simulink model "HSX_PPS_series0226_2"  (R2023b)
settings: Solver=VariableStepAuto  StartTime=0.0  StopTime=10  RelTol=1e-3
undefined symbols (not defined in the file): Kanti, Ki, Kp, LHSX, Ra, RHSX, Tsamp, Vf
libraries: spsVoltageMeasurementLib x39, spsControlledVoltageSourceLib x32, spsDCMachineLib x32, spsSeriesRLCBranchLib x8, spsCurrentMeasurementLib x6, spsGroundLib x3, spsIdealSwitchLib x2, spsMosfetLib x2, spsPWMGenerator2LevelLib x1, spsDCVoltageSourceLib x1, spsDiodeLib x1, spsVariableRatioTransformerLib x1
(part 1 of 2)
settings Model: Creator=Hyeongmeen  LastModifiedBy=Hyeongmeen

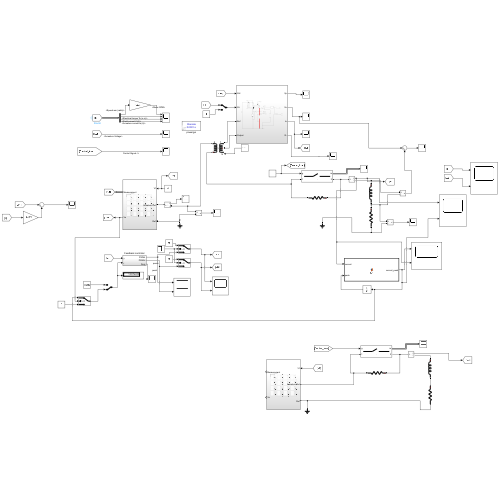
[thumbnail: Simulink's stored preview of the top-level diagram]
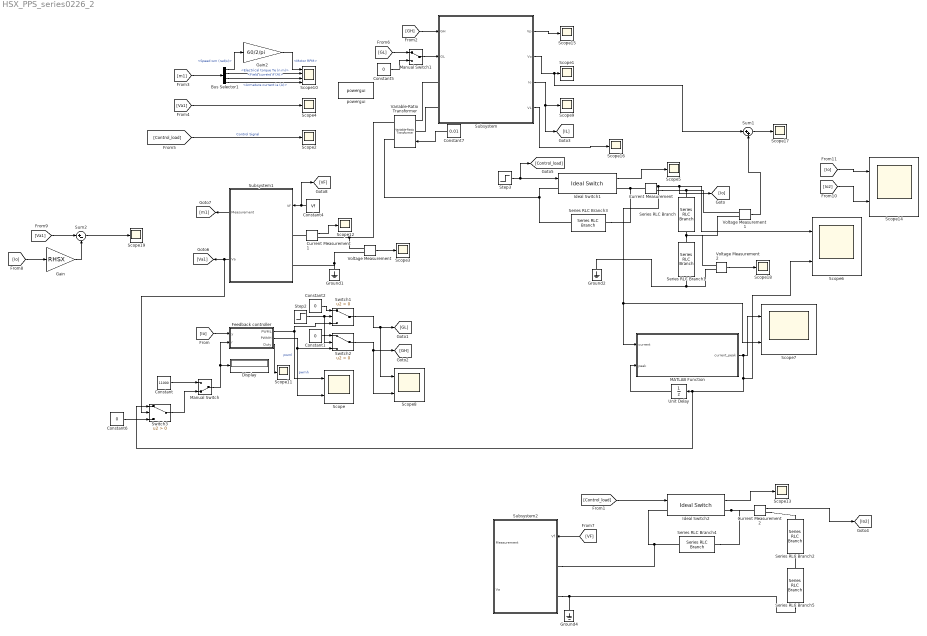
== system HSX_PPS_series0226_2 ==
  Bus Selector1 : BusSelector  OutputSignals=Speed wm (rad/s),Electrical torque Te (n m),Field current if (A),Armature current ia (A)
  Constant : Constant  Value=11000
  Constant{1..2,5..6} (4 alike) : Constant  Value=0
  Constant4 : Constant  Value=Vf
  Constant7 : Constant  Value=0.01
  Current Measurement : spsCurrentMeasurementLib/Current Measurement  PhasorSimulation=off  OutputType=Complex  PSBequivalent=0
  Current Measurement1 : spsCurrentMeasurementLib/Current Measurement  PhasorSimulation=off  OutputType=Complex  PSBequivalent=0
  Current Measurement2 : spsCurrentMeasurementLib/Current Measurement  PhasorSimulation=off  OutputType=Complex  PSBequivalent=0
  Display : Display
  Feedback controller : Subsystem
  Gain : Gain  Gain=RHSX
  Gain2 : Gain  Gain=60/2/pi
  Ground1 : spsGroundLib/Ground  LConnTagsString=a
  Ground2 : spsGroundLib/Ground  LConnTagsString=a
  Ground4 : spsGroundLib/Ground  LConnTagsString=a
  Ideal Switch1 : spsIdealSwitchLib/Ideal Switch  Ron=0.01  Lon=0  IC=0  Rs=1e6  Cs=0  Measurements=on
  Ideal Switch2 : spsIdealSwitchLib/Ideal Switch  Ron=0.01  Lon=0  IC=0  Rs=1e6  Cs=0  Measurements=on
  MATLAB Function : MATLAB Function  TreatAsAtomicUnit=on
  Manual Switch : ManualSwitch  CurrentSetting=0
  Manual Switch1 : ManualSwitch
  Scope{,6..8,14} (5 alike) : Scope  NumInputPorts=2
  Scope{1..5,9,11..13,15..19} (14 alike) : Scope
  Scope10 : Scope  NumInputPorts=4
  Series RLC Branch : spsSeriesRLCBranchLib/Series RLC Branch  LConnTagsString=__new0  RConnTagsString=__new0  BranchType=L  Resistance=RHSX  Inductance=LHSX  SetiL0=off  InitialCurrent=0  Capacitance=1e-6  Setx0=off  InitialVoltage=0  Measurements=None
  Series RLC Branch1 : spsSeriesRLCBranchLib/Series RLC Branch  LConnTagsString=__new0  RConnTagsString=__new0  BranchType=R  Resistance=RHSX  Inductance=LHSX  SetiL0=off  InitialCurrent=0  Capacitance=1e-6  Setx0=off  InitialVoltage=0  Measurements=None
  Series RLC Branch2 : spsSeriesRLCBranchLib/Series RLC Branch  LConnTagsString=__new0  RConnTagsString=__new0  BranchType=L  Resistance=RHSX  Inductance=LHSX  SetiL0=off  InitialCurrent=0  Capacitance=1e-6  Setx0=off  InitialVoltage=0  Measurements=None
  Series RLC Branch3 : spsSeriesRLCBranchLib/Series RLC Branch  LConnTagsString=__new0  RConnTagsString=__new0  BranchType=R  Resistance=1e8  Inductance=0  SetiL0=off  InitialCurrent=0  Capacitance=1e-6  Setx0=off  InitialVoltage=0  Measurements=None
  Series RLC Branch4 : spsSeriesRLCBranchLib/Series RLC Branch  LConnTagsString=__new0  RConnTagsString=__new0  BranchType=R  Resistance=1e8  Inductance=0  SetiL0=off  InitialCurrent=0  Capacitance=1e-6  Setx0=off  InitialVoltage=0  Measurements=None
  Series RLC Branch5 : spsSeriesRLCBranchLib/Series RLC Branch  LConnTagsString=__new0  RConnTagsString=__new0  BranchType=R  Resistance=RHSX  Inductance=LHSX  SetiL0=off  InitialCurrent=0  Capacitance=1e-6  Setx0=off  InitialVoltage=0  Measurements=None
  Step2 : Step  Time=5  Before=1  After=0  SampleTime=0  VectorParams1D=off  ZeroCross=off
  Step3 : Step  Time=5  SampleTime=0  VectorParams1D=off  ZeroCross=off
  Subsystem : Subsystem
  Subsystem1 : Subsystem
  Subsystem2 : Subsystem
  Sum1 : Sum  Inputs=|++
  Sum2 : Sum  Inputs=|+-
  Switch1 : Switch  Criteria=u2 > Threshold  SaturateOnIntegerOverflow=off  InputSameDT=off
  Switch2 : Switch  Criteria=u2 > Threshold  SaturateOnIntegerOverflow=off  InputSameDT=off
  Switch3 : Switch  Criteria=u2 > Threshold  SaturateOnIntegerOverflow=off  InputSameDT=off
  Unit Delay : UnitDelay  SampleTime=-1  HasFrameUpgradeWarning=on
  Variable-Ratio Transformer : spsVariableRatioTransformerLib/Variable-Ratio Transformer
      settings: LibrarySourceBlock=|
      | sps_lib/Passives/Variable-Ratio
      | Transformer
  Voltage Measurement : spsVoltageMeasurementLib/Voltage Measurement  PhasorSimulation=off  OutputType=Complex  PSBequivalent=0
  Voltage Measurement1 : spsVoltageMeasurementLib/Voltage Measurement  PhasorSimulation=off  OutputType=Complex  PSBequivalent=0
  Voltage Measurement2 : spsVoltageMeasurementLib/Voltage Measurement  PhasorSimulation=off  OutputType=Complex  PSBequivalent=0
  powergui : sps_lib/powergui  Priority=1  SimulationMode=Discrete  SampleTime=Tsamp  frequency=60  Iterations=50  frequencyindice=0  Pbase=100e6  ErrMax=1e-4  UnitsV=kV  UnitsW=MW  buscounter=0  FunctionMessages=off  echomessages=off  EnableUseOfTLC=off  CurrentSourceSwitches=off  DisableSnubberDevices=off  DisableRonSwitches=off  DisableVfSwitches=off  DisplayEquations=off  AutomaticDiscreteSolvers=off  SolverType=Tustin/Backward Euler (TBE)  Interpol=off  ExternalGateDelay=off  methode=off  Ts=100  x0status=blocks  SPID=on  SwTol=0  HookPort=off  NonlinearTolerance=1e-4  nMaxIteration=100  ContinueOnMaxIteration=off  RestoreLinks=warning  ResistiveCurrentMeasurement=off  Frange=[0:2:500]  Ylog=off  Xlog=on  ShowGrid=off  save=off  variable=ZData  structure=0  ZoomFFT=off  StartTime=0.0  cycles=1  DisplayStyle=1  fundamental=60  FreqAxis=off  MaxFrequency=1000  frequencyindicesteady=1  RmsSteady=1  display=off
  wires:
  Bus Selector1/1 -> Gain2/1  "<Speed wm (rad/s)>"
  Bus Selector1/4 -> Scope10/4  "<Armature current ia (A)>"
  Bus Selector1/2 -> Scope10/2  "<Electrical torque Te (n m)>"
  Gain2/1 -> Scope10/1  "<Motor RPM>"
  Bus Selector1/3 -> Scope10/3  "<Field current if (A)>"
  [m1] -> Bus Selector1/1
  Step3/1 -> [Control_load], Ideal Switch1/1
  Step2/1 -> Switch2/2, Switch1/2
  Feedback controller/2(PWMH) -> Switch2/3, Scope/2  "pwmh"
  Feedback controller/1(PWML) -> Scope/1, Switch1/3  "pwml"
  Constant2/1 -> Switch1/1
  Constant1/1 -> Switch2/1
  [Control_load] -> Scope2/1  "Control Signal"
  [Va1] -> Scope4/1
  Subsystem1/2(Va) -> Switch3/2, [Va1]
  Subsystem1/1(Measurement) -> [m1]
  Constant4/1 -> [VF], Subsystem1/1(Vf)
  Ideal Switch1/1 -> Scope5/1
  Current Measurement/1 -> Scope7/2, MATLAB Function/1(current), [Io], Scope6/1
  Unit Delay/1 -> MATLAB Function/2(peak)
  Switch1/1 -> Scope8/1, [GL]
  Switch2/1 -> Scope8/2, [GH]
  Subsystem/2(Vo) -> Sum1/1, Scope1/1
  Voltage Measurement/1 -> Scope3/1
  Subsystem/3(Io) -> [IL], Scope9/1
  Manual Switch1/1 -> Subsystem/2(GL)
  [Io] -> Feedback controller/1(y)
  Feedback controller/3(Duty) -> Scope11/1
  Constant/1 -> Manual Switch/1
  Manual Switch/1 -> Display/1, Feedback controller/2(r)
  [GH] -> Subsystem/1(GH)
  [GL] -> Manual Switch1/1
  Constant5/1 -> Manual Switch1/2
  MATLAB Function/1(current_peak) -> Scope6/2, Switch3/1, Unit Delay/1, Scope7/1
  Switch3/1 -> Manual Switch/2
  Constant6/1 -> Switch3/3
  Subsystem/1(Vp) -> Scope15/1
  Subsystem/4(VL) -> Scope16/1
  Voltage Measurement1/1 -> Sum1/2
  Sum1/1 -> Scope17/1
  Voltage Measurement2/1 -> Scope18/1
  [Va1] -> Sum2/1
  [Io] -> Gain/1
  Gain/1 -> Sum2/2
  Sum2/1 -> Scope19/1
  Current Measurement1/1 -> Scope12/1
  Constant7/1 -> Variable-Ratio Transformer/1
  Ideal Switch2/1 -> Scope13/1
  [Control_load] -> Ideal Switch2/1
  [VF] -> Subsystem2/1(Vf)
  Current Measurement2/1 -> [Io2]
  [Io] -> Scope14/1
  [Io2] -> Scope14/2
  connections:
  Series RLC Branch3/LConn1 -- Current Measurement/LConn1 -- Ideal Switch1/RConn1
  Ground1/LConn1 -- Voltage Measurement/LConn2 -- Subsystem1/LConn2
  Current Measurement/RConn1 -- Voltage Measurement1/LConn1 -- Series RLC Branch/LConn1
  Voltage Measurement/LConn1 -- Variable-Ratio Transformer/RConn2 -- Current Measurement1/RConn1
  Ground2/LConn1 -- Voltage Measurement2/LConn2 -- Series RLC Branch1/RConn1
  Series RLC Branch/RConn1 -- Voltage Measurement2/LConn1 -- Voltage Measurement1/LConn2 -- Series RLC Branch1/LConn1
  Subsystem/LConn1 -- Variable-Ratio Transformer/LConn2
  Current Measurement1/LConn1 -- Subsystem1/LConn1
  Ideal Switch1/LConn1 -- Variable-Ratio Transformer/RConn1 -- Series RLC Branch3/RConn1
  Subsystem/LConn2 -- Variable-Ratio Transformer/LConn1
  Ideal Switch2/LConn1 -- Subsystem2/LConn1 -- Series RLC Branch4/RConn1
  Current Measurement2/RConn1 -- Series RLC Branch2/LConn1
  Ideal Switch2/RConn1 -- Series RLC Branch4/LConn1 -- Current Measurement2/LConn1
  Subsystem2/LConn2 -- Series RLC Branch5/RConn1 -- Ground4/LConn1
  Series RLC Branch5/LConn1 -- Series RLC Branch2/RConn1

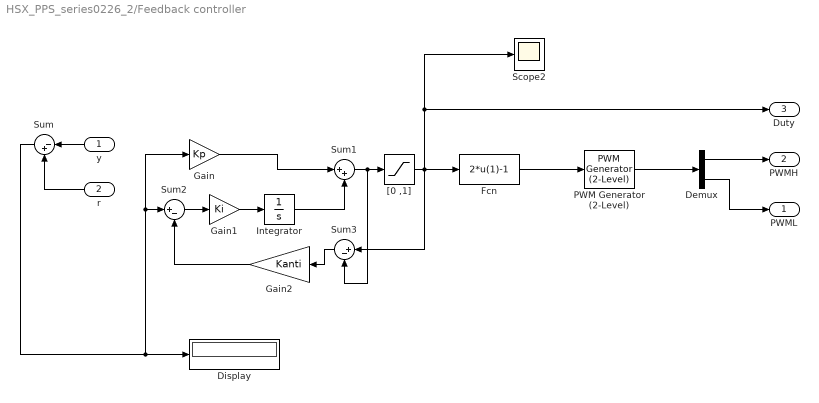
== system HSX_PPS_series0226_2/Feedback controller ==
  y : Inport
  r : Inport  Port=2
  Demux : Demux  Outputs=2
  Display : Display
  Fcn : Fcn  Expr=2*u(1)-1
  Gain : Gain  Gain=Kp
  Gain1 : Gain  Gain=Ki
  Gain2 : Gain  Gain=Kanti
  Integrator : Integrator
  PWM Generator (2-Level) : spsPWMGenerator2LevelLib/PWM Generator (2-Level)  ModulatorType=Single-phase half-bridge (2 pulses)  ModulatorMode=Unsynchronized  Fc=10000  Pc=90  nF=27  MinMax="[ -1  1 ]"  SamplingTechnique=Natural  ModulatingSignals=off  m=0.8  Freq=60  Phase=0  Ts=0  ShowCarrierOutport=off
  Scope2 : Scope
  Sum : Sum  Inputs=|-+  InputSameDT=on  SaturateOnIntegerOverflow=on  OutDataTypeStr=Inherit: Same as first input
  Sum1 : Sum  Inputs=|++
  Sum2 : Sum  Inputs=|+-
  Sum3 : Sum  Inputs=|+-
  "[0 ,1]" : Saturate  UpperLimit=1  LowerLimit=0
  PWML : Outport  VectorParamsAs1DForOutWhenUnconnected=off
  PWMH : Outport  Port=2  VectorParamsAs1DForOutWhenUnconnected=off
  Duty : Outport  Port=3  VectorParamsAs1DForOutWhenUnconnected=off
  wires:
  Sum/1 -> Display/1, Gain/1, Sum2/1
  y/1 -> Sum/1
  r/1 -> Sum/2
  "[0 ,1]"/1 -> Sum3/1, Fcn/1, Scope2/1, Duty/1
  Fcn/1 -> PWM Generator (2-Level)/1
  PWM Generator (2-Level)/1 -> Demux/1
  Demux/1 -> PWMH/1
  Demux/2 -> PWML/1
  Gain1/1 -> Integrator/1
  Sum1/1 -> Sum3/2, "[0 ,1]"/1
  Gain/1 -> Sum1/1
  Integrator/1 -> Sum1/2
  Sum2/1 -> Gain1/1
  Sum3/1 -> Gain2/1
  Gain2/1 -> Sum2/2

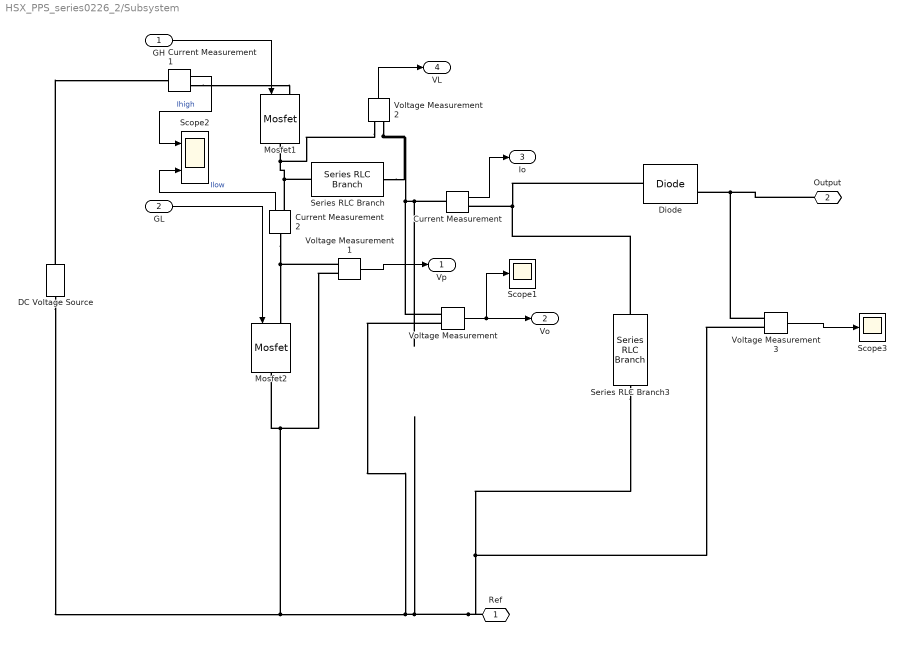
== system HSX_PPS_series0226_2/Subsystem ==
  GH : Inport
  GL : Inport  Port=2
  Current Measurement : spsCurrentMeasurementLib/Current Measurement  PhasorSimulation=off  OutputType=Complex  PSBequivalent=0
  Current Measurement1 : spsCurrentMeasurementLib/Current Measurement  PhasorSimulation=off  OutputType=Complex  PSBequivalent=0
  Current Measurement2 : spsCurrentMeasurementLib/Current Measurement  PhasorSimulation=off  OutputType=Complex  PSBequivalent=0
  DC Voltage Source : spsDCVoltageSourceLib/DC Voltage Source  Amplitude=2000  Measurements=None
  Diode : spsDiodeLib/Diode  Ron=0.001  Lon=0  Vf=0.8  IC=0  UseSnubber=0  Rs=500  Cs=250e-9  Measurements=on
  Mosfet1 : spsMosfetLib/Mosfet  Ron=0.00001  Lon=0  Rd=0.01  Vfd=0.8  IC=0  Rs=1e5  Cs=inf  Measurements=off
  Mosfet2 : spsMosfetLib/Mosfet  Ron=0.00001  Lon=0  Rd=0.01  Vfd=0.8  IC=0  Rs=1e5  Cs=inf  Measurements=off
  Scope1 : Scope
  Scope2 : Scope  NumInputPorts=2
  Scope3 : Scope
  Series RLC Branch : spsSeriesRLCBranchLib/Series RLC Branch  LConnTagsString=__new0  RConnTagsString=__new0  BranchType=L  Resistance=RHSX  Inductance=0.0001  SetiL0=off  InitialCurrent=0  Capacitance=1e-6  Setx0=off  InitialVoltage=0  Measurements=None
  Series RLC Branch3 : spsSeriesRLCBranchLib/Series RLC Branch  LConnTagsString=__new0  RConnTagsString=__new0  BranchType=R  Resistance=1e8  Inductance=0  SetiL0=off  InitialCurrent=0  Capacitance=1e-6  Setx0=off  InitialVoltage=0  Measurements=None
  Voltage Measurement{,1..3} (4 alike) : spsVoltageMeasurementLib/Voltage Measurement  PhasorSimulation=off  OutputType=Complex  PSBequivalent=0
  Ref : PMIOPort  Side=Left
  Output : PMIOPort  Port=2  Side=Left
  Vp : Outport
  Vo : Outport  Port=2
  Io : Outport  Port=3
  VL : Outport  Port=4
  wires:
  Voltage Measurement/1 -> Vo/1, Scope1/1
  Voltage Measurement1/1 -> Vp/1
  GL/1 -> Mosfet2/1
  GH/1 -> Mosfet1/1
  Current Measurement/1 -> Io/1
  Current Measurement1/1 -> Scope2/1  "Ihigh"
  Current Measurement2/1 -> Scope2/2  "Ilow"
  Voltage Measurement2/1 -> VL/1
  Voltage Measurement3/1 -> Scope3/1
  connections:
  Current Measurement2/RConn1 -- Series RLC Branch/LConn1 -- Voltage Measurement2/LConn1 -- Mosfet1/RConn1
  Ref/RConn1 -- Voltage Measurement3/LConn2 -- Series RLC Branch3/LConn1 -- Voltage Measurement/LConn2 -- Voltage Measurement1/LConn2 -- Mosfet2/RConn1 -- DC Voltage Source/LConn1
  Series RLC Branch3/RConn1 -- Diode/LConn1 -- Current Measurement/RConn1
  DC Voltage Source/RConn1 -- Current Measurement1/LConn1
  Current Measurement1/RConn1 -- Mosfet1/LConn1
  Voltage Measurement1/LConn1 -- Current Measurement2/LConn1 -- Mosfet2/LConn1
  Voltage Measurement2/LConn2 -- Series RLC Branch/RConn1 -- Voltage Measurement/LConn1 -- Current Measurement/LConn1
  Output/RConn1 -- Voltage Measurement3/LConn1 -- Diode/RConn1

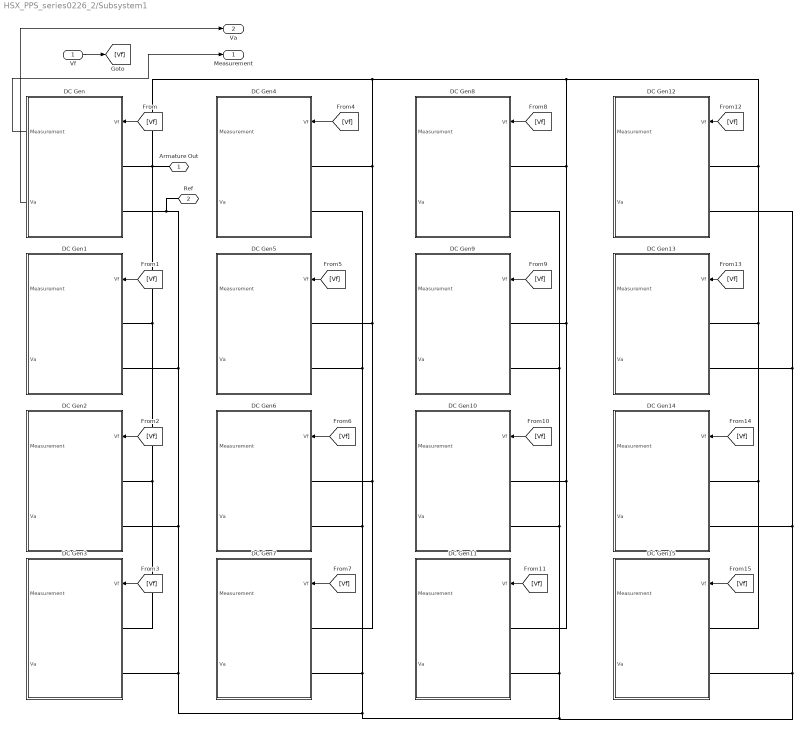
== system HSX_PPS_series0226_2/Subsystem1 ==
  Vf : Inport
  DC Gen : Subsystem
  DC Gen1 : Subsystem
  DC Gen10 : Subsystem
  DC Gen11 : Subsystem
  DC Gen12 : Subsystem
  DC Gen13 : Subsystem
  DC Gen14 : Subsystem
  DC Gen15 : Subsystem
  DC Gen2 : Subsystem
  DC Gen3 : Subsystem
  DC Gen4 : Subsystem
  DC Gen5 : Subsystem
  DC Gen6 : Subsystem
  DC Gen7 : Subsystem
  DC Gen8 : Subsystem
  DC Gen9 : Subsystem
  Armature Out : PMIOPort  Side=Left
  Ref : PMIOPort  Port=2  Side=Left
  Measurement : Outport
  Va : Outport  Port=2
  wires:
  Vf/1 -> [Vf]
  [Vf] -> DC Gen/1(Vf)
  [Vf] -> DC Gen1/1(Vf)
  [Vf] -> DC Gen2/1(Vf)
  [Vf] -> DC Gen3/1(Vf)
  [Vf] -> DC Gen4/1(Vf)
  [Vf] -> DC Gen5/1(Vf)
  [Vf] -> DC Gen6/1(Vf)
  [Vf] -> DC Gen7/1(Vf)
  [Vf] -> DC Gen8/1(Vf)
  [Vf] -> DC Gen9/1(Vf)
  [Vf] -> DC Gen10/1(Vf)
  [Vf] -> DC Gen11/1(Vf)
  [Vf] -> DC Gen12/1(Vf)
  [Vf] -> DC Gen13/1(Vf)
  [Vf] -> DC Gen14/1(Vf)
  [Vf] -> DC Gen15/1(Vf)
  DC Gen/1(Measurement) -> Measurement/1
  DC Gen/2(Va) -> Va/1
  connections:
  DC Gen11/LConn1 -- DC Gen10/LConn1 -- DC Gen9/LConn1 -- DC Gen8/LConn1 -- DC Gen7/LConn1 -- DC Gen6/LConn1 -- DC Gen5/LConn1 -- DC Gen4/LConn1 -- DC Gen1/LConn1 -- DC Gen2/LConn1 -- DC Gen3/LConn1 -- DC Gen/LConn1 -- Armature Out/RConn1 -- DC Gen12/LConn1 -- DC Gen13/LConn1 -- DC Gen14/LConn1 -- DC Gen15/LConn1
  DC Gen8/LConn2 -- DC Gen9/LConn2 -- DC Gen10/LConn2 -- DC Gen11/LConn2 -- DC Gen4/LConn2 -- DC Gen5/LConn2 -- DC Gen6/LConn2 -- DC Gen7/LConn2 -- DC Gen3/LConn2 -- DC Gen1/LConn2 -- Ref/RConn1 -- DC Gen/LConn2 -- DC Gen2/LConn2 -- DC Gen15/LConn2 -- DC Gen12/LConn2 -- DC Gen13/LConn2 -- DC Gen14/LConn2

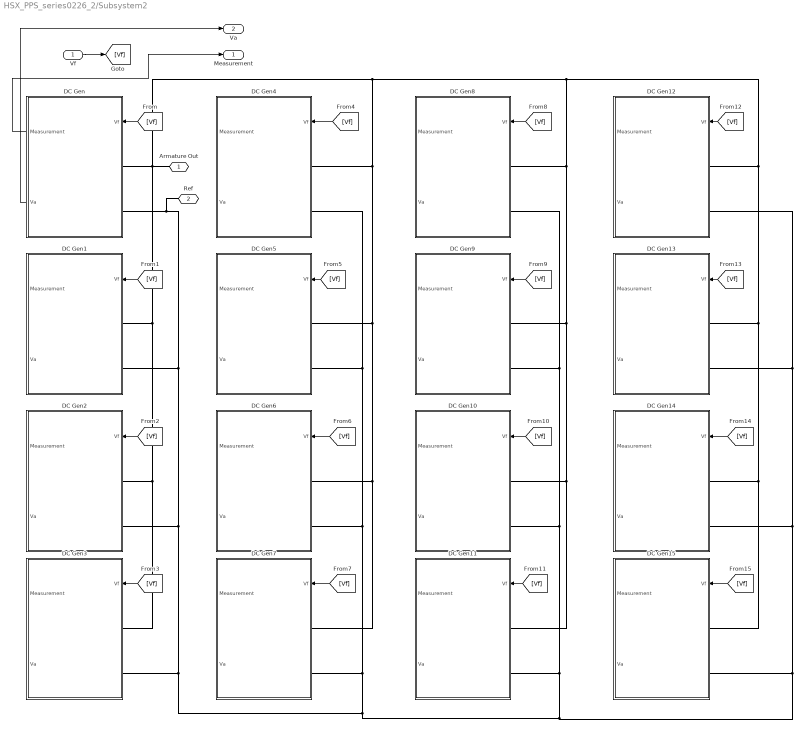
== system HSX_PPS_series0226_2/Subsystem2 ==
  Vf : Inport
  DC Gen : Subsystem
  DC Gen1 : Subsystem
  DC Gen10 : Subsystem
  DC Gen11 : Subsystem
  DC Gen12 : Subsystem
  DC Gen13 : Subsystem
  DC Gen14 : Subsystem
  DC Gen15 : Subsystem
  DC Gen2 : Subsystem
  DC Gen3 : Subsystem
  DC Gen4 : Subsystem
  DC Gen5 : Subsystem
  DC Gen6 : Subsystem
  DC Gen7 : Subsystem
  DC Gen8 : Subsystem
  DC Gen9 : Subsystem
  Armature Out : PMIOPort  Side=Left
  Ref : PMIOPort  Port=2  Side=Left
  Measurement : Outport
  Va : Outport  Port=2
  wires:
  Vf/1 -> [Vf]
  [Vf] -> DC Gen/1(Vf)
  [Vf] -> DC Gen1/1(Vf)
  [Vf] -> DC Gen2/1(Vf)
  [Vf] -> DC Gen3/1(Vf)
  [Vf] -> DC Gen4/1(Vf)
  [Vf] -> DC Gen5/1(Vf)
  [Vf] -> DC Gen6/1(Vf)
  [Vf] -> DC Gen7/1(Vf)
  [Vf] -> DC Gen8/1(Vf)
  [Vf] -> DC Gen9/1(Vf)
  [Vf] -> DC Gen10/1(Vf)
  [Vf] -> DC Gen11/1(Vf)
  [Vf] -> DC Gen12/1(Vf)
  [Vf] -> DC Gen13/1(Vf)
  [Vf] -> DC Gen14/1(Vf)
  [Vf] -> DC Gen15/1(Vf)
  DC Gen/1(Measurement) -> Measurement/1
  DC Gen/2(Va) -> Va/1
  connections:
  DC Gen11/LConn1 -- DC Gen10/LConn1 -- DC Gen9/LConn1 -- DC Gen8/LConn1 -- DC Gen7/LConn1 -- DC Gen6/LConn1 -- DC Gen5/LConn1 -- DC Gen4/LConn1 -- DC Gen1/LConn1 -- DC Gen2/LConn1 -- DC Gen3/LConn1 -- DC Gen/LConn1 -- Armature Out/RConn1 -- DC Gen12/LConn1 -- DC Gen13/LConn1 -- DC Gen14/LConn1 -- DC Gen15/LConn1
  DC Gen8/LConn2 -- DC Gen9/LConn2 -- DC Gen10/LConn2 -- DC Gen11/LConn2 -- DC Gen4/LConn2 -- DC Gen5/LConn2 -- DC Gen6/LConn2 -- DC Gen7/LConn2 -- DC Gen3/LConn2 -- DC Gen1/LConn2 -- Ref/RConn1 -- DC Gen/LConn2 -- DC Gen2/LConn2 -- DC Gen15/LConn2 -- DC Gen12/LConn2 -- DC Gen13/LConn2 -- DC Gen14/LConn2

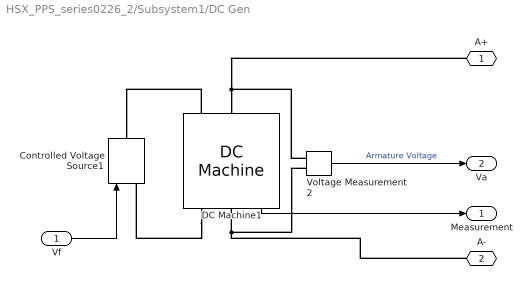
== system HSX_PPS_series0226_2/Subsystem1/DC Gen ==
  Vf : Inport
  Controlled Voltage Source1 : spsControlledVoltageSourceLib/Controlled Voltage Source  Initialize=on  Source_Type=DC  Amplitude=0  Phase=0  Frequency=0  Measurements=Voltage
  DC Machine1 : spsDCMachineLib/DC Machine  PresetModel=No  MechanicalLoad=Torque TL  FieldType=Wound  ShowDetailedParameters=on  MeasurementBus=off  RLa="[Ra  0.002]"  RLf=[0.0054 0.0125]  Laf=Laf  MachineConstant=Torque constant (N.m/A)  Ke=1.8  Kt=1.8  J=137  Bm=0  Tf=0  w0=w_initial  Ifinit=0  TsPowergui=0  TsBlock=-1
  Voltage Measurement2 : spsVoltageMeasurementLib/Voltage Measurement  PhasorSimulation=off  OutputType=Complex  PSBequivalent=0
  A+ : PMIOPort  Side=Left
  A- : PMIOPort  Port=2  Side=Left
  Measurement : Outport
  Va : Outport  Port=2
  wires:
  DC Machine1/1 -> Measurement/1
  Vf/1 -> Controlled Voltage Source1/1
  Voltage Measurement2/1 -> Va/1  "Armature Voltage"
  connections:
  Voltage Measurement2/LConn1 -- A+/RConn1 -- DC Machine1/LConn1
  A-/RConn1 -- Voltage Measurement2/LConn2 -- DC Machine1/RConn1
  DC Machine1/LConn2 -- Controlled Voltage Source1/RConn1
  DC Machine1/RConn2 -- Controlled Voltage Source1/LConn1

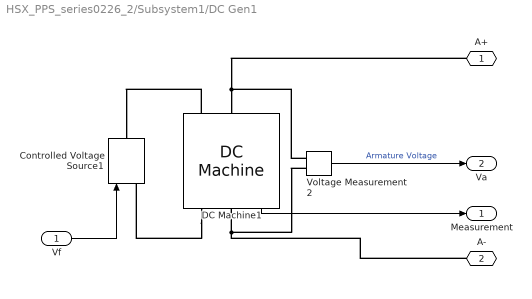
== system HSX_PPS_series0226_2/Subsystem1/DC Gen1 ==
  Vf : Inport
  Controlled Voltage Source1 : spsControlledVoltageSourceLib/Controlled Voltage Source  Initialize=on  Source_Type=DC  Amplitude=0  Phase=0  Frequency=0  Measurements=Voltage
  DC Machine1 : spsDCMachineLib/DC Machine  PresetModel=No  MechanicalLoad=Torque TL  FieldType=Wound  ShowDetailedParameters=on  MeasurementBus=off  RLa="[Ra  0.002]"  RLf=[0.0054 0.0125]  Laf=Laf  MachineConstant=Torque constant (N.m/A)  Ke=1.8  Kt=1.8  J=137  Bm=0  Tf=0  w0=w_initial  Ifinit=0  TsPowergui=0  TsBlock=-1
  Voltage Measurement2 : spsVoltageMeasurementLib/Voltage Measurement  PhasorSimulation=off  OutputType=Complex  PSBequivalent=0
  A+ : PMIOPort  Side=Left
  A- : PMIOPort  Port=2  Side=Left
  Measurement : Outport
  Va : Outport  Port=2
  wires:
  DC Machine1/1 -> Measurement/1
  Vf/1 -> Controlled Voltage Source1/1
  Voltage Measurement2/1 -> Va/1  "Armature Voltage"
  connections:
  Voltage Measurement2/LConn1 -- A+/RConn1 -- DC Machine1/LConn1
  A-/RConn1 -- Voltage Measurement2/LConn2 -- DC Machine1/RConn1
  DC Machine1/LConn2 -- Controlled Voltage Source1/RConn1
  DC Machine1/RConn2 -- Controlled Voltage Source1/LConn1

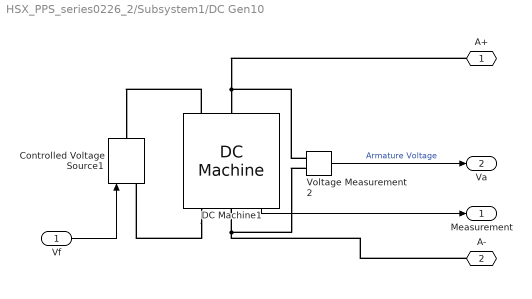
== system HSX_PPS_series0226_2/Subsystem1/DC Gen10 ==
  Vf : Inport
  Controlled Voltage Source1 : spsControlledVoltageSourceLib/Controlled Voltage Source  Initialize=on  Source_Type=DC  Amplitude=0  Phase=0  Frequency=0  Measurements=Voltage
  DC Machine1 : spsDCMachineLib/DC Machine  PresetModel=No  MechanicalLoad=Torque TL  FieldType=Wound  ShowDetailedParameters=on  MeasurementBus=off  RLa="[Ra  0.002]"  RLf=[0.0054 0.0125]  Laf=Laf  MachineConstant=Torque constant (N.m/A)  Ke=1.8  Kt=1.8  J=137  Bm=0  Tf=0  w0=w_initial  Ifinit=0  TsPowergui=0  TsBlock=-1
  Voltage Measurement2 : spsVoltageMeasurementLib/Voltage Measurement  PhasorSimulation=off  OutputType=Complex  PSBequivalent=0
  A+ : PMIOPort  Side=Left
  A- : PMIOPort  Port=2  Side=Left
  Measurement : Outport
  Va : Outport  Port=2
  wires:
  DC Machine1/1 -> Measurement/1
  Vf/1 -> Controlled Voltage Source1/1
  Voltage Measurement2/1 -> Va/1  "Armature Voltage"
  connections:
  Voltage Measurement2/LConn1 -- A+/RConn1 -- DC Machine1/LConn1
  A-/RConn1 -- Voltage Measurement2/LConn2 -- DC Machine1/RConn1
  DC Machine1/LConn2 -- Controlled Voltage Source1/RConn1
  DC Machine1/RConn2 -- Controlled Voltage Source1/LConn1

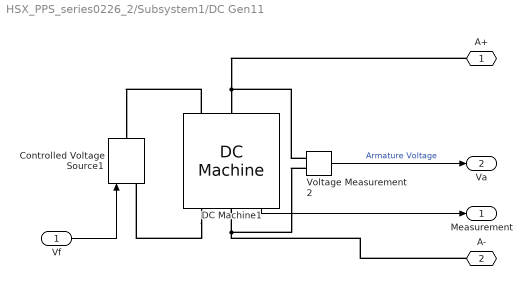
== system HSX_PPS_series0226_2/Subsystem1/DC Gen11 ==
  Vf : Inport
  Controlled Voltage Source1 : spsControlledVoltageSourceLib/Controlled Voltage Source  Initialize=on  Source_Type=DC  Amplitude=0  Phase=0  Frequency=0  Measurements=Voltage
  DC Machine1 : spsDCMachineLib/DC Machine  PresetModel=No  MechanicalLoad=Torque TL  FieldType=Wound  ShowDetailedParameters=on  MeasurementBus=off  RLa="[Ra  0.002]"  RLf=[0.0054 0.0125]  Laf=Laf  MachineConstant=Torque constant (N.m/A)  Ke=1.8  Kt=1.8  J=137  Bm=0  Tf=0  w0=w_initial  Ifinit=0  TsPowergui=0  TsBlock=-1
  Voltage Measurement2 : spsVoltageMeasurementLib/Voltage Measurement  PhasorSimulation=off  OutputType=Complex  PSBequivalent=0
  A+ : PMIOPort  Side=Left
  A- : PMIOPort  Port=2  Side=Left
  Measurement : Outport
  Va : Outport  Port=2
  wires:
  DC Machine1/1 -> Measurement/1
  Vf/1 -> Controlled Voltage Source1/1
  Voltage Measurement2/1 -> Va/1  "Armature Voltage"
  connections:
  Voltage Measurement2/LConn1 -- A+/RConn1 -- DC Machine1/LConn1
  A-/RConn1 -- Voltage Measurement2/LConn2 -- DC Machine1/RConn1
  DC Machine1/LConn2 -- Controlled Voltage Source1/RConn1
  DC Machine1/RConn2 -- Controlled Voltage Source1/LConn1

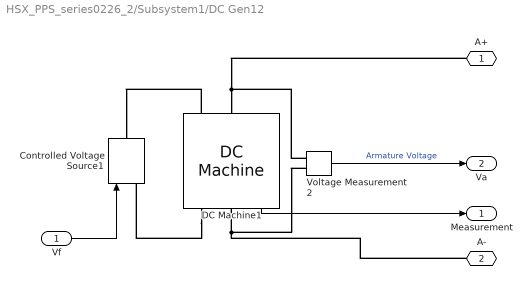
== system HSX_PPS_series0226_2/Subsystem1/DC Gen12 ==
  Vf : Inport
  Controlled Voltage Source1 : spsControlledVoltageSourceLib/Controlled Voltage Source  Initialize=on  Source_Type=DC  Amplitude=0  Phase=0  Frequency=0  Measurements=Voltage
  DC Machine1 : spsDCMachineLib/DC Machine  PresetModel=No  MechanicalLoad=Torque TL  FieldType=Wound  ShowDetailedParameters=on  MeasurementBus=off  RLa="[Ra  0.002]"  RLf=[0.0054 0.0125]  Laf=Laf  MachineConstant=Torque constant (N.m/A)  Ke=1.8  Kt=1.8  J=137  Bm=0  Tf=0  w0=w_initial  Ifinit=0  TsPowergui=0  TsBlock=-1
  Voltage Measurement2 : spsVoltageMeasurementLib/Voltage Measurement  PhasorSimulation=off  OutputType=Complex  PSBequivalent=0
  A+ : PMIOPort  Side=Left
  A- : PMIOPort  Port=2  Side=Left
  Measurement : Outport
  Va : Outport  Port=2
  wires:
  DC Machine1/1 -> Measurement/1
  Vf/1 -> Controlled Voltage Source1/1
  Voltage Measurement2/1 -> Va/1  "Armature Voltage"
  connections:
  Voltage Measurement2/LConn1 -- A+/RConn1 -- DC Machine1/LConn1
  A-/RConn1 -- Voltage Measurement2/LConn2 -- DC Machine1/RConn1
  DC Machine1/LConn2 -- Controlled Voltage Source1/RConn1
  DC Machine1/RConn2 -- Controlled Voltage Source1/LConn1

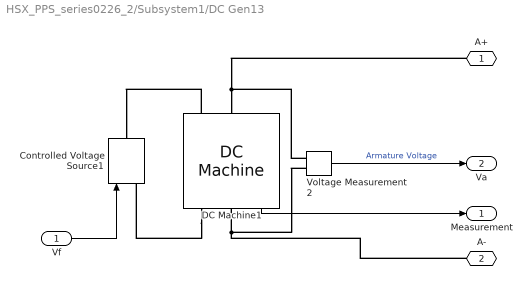
== system HSX_PPS_series0226_2/Subsystem1/DC Gen13 ==
  Vf : Inport
  Controlled Voltage Source1 : spsControlledVoltageSourceLib/Controlled Voltage Source  Initialize=on  Source_Type=DC  Amplitude=0  Phase=0  Frequency=0  Measurements=Voltage
  DC Machine1 : spsDCMachineLib/DC Machine  PresetModel=No  MechanicalLoad=Torque TL  FieldType=Wound  ShowDetailedParameters=on  MeasurementBus=off  RLa="[Ra  0.002]"  RLf=[0.0054 0.0125]  Laf=Laf  MachineConstant=Torque constant (N.m/A)  Ke=1.8  Kt=1.8  J=137  Bm=0  Tf=0  w0=w_initial  Ifinit=0  TsPowergui=0  TsBlock=-1
  Voltage Measurement2 : spsVoltageMeasurementLib/Voltage Measurement  PhasorSimulation=off  OutputType=Complex  PSBequivalent=0
  A+ : PMIOPort  Side=Left
  A- : PMIOPort  Port=2  Side=Left
  Measurement : Outport
  Va : Outport  Port=2
  wires:
  DC Machine1/1 -> Measurement/1
  Vf/1 -> Controlled Voltage Source1/1
  Voltage Measurement2/1 -> Va/1  "Armature Voltage"
  connections:
  Voltage Measurement2/LConn1 -- A+/RConn1 -- DC Machine1/LConn1
  A-/RConn1 -- Voltage Measurement2/LConn2 -- DC Machine1/RConn1
  DC Machine1/LConn2 -- Controlled Voltage Source1/RConn1
  DC Machine1/RConn2 -- Controlled Voltage Source1/LConn1

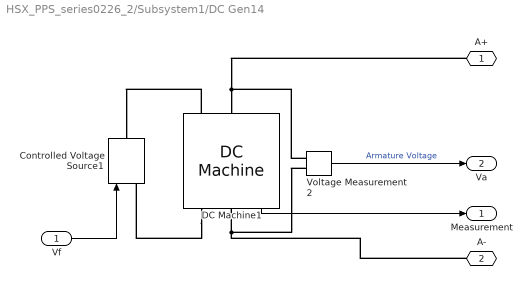
== system HSX_PPS_series0226_2/Subsystem1/DC Gen14 ==
  Vf : Inport
  Controlled Voltage Source1 : spsControlledVoltageSourceLib/Controlled Voltage Source  Initialize=on  Source_Type=DC  Amplitude=0  Phase=0  Frequency=0  Measurements=Voltage
  DC Machine1 : spsDCMachineLib/DC Machine  PresetModel=No  MechanicalLoad=Torque TL  FieldType=Wound  ShowDetailedParameters=on  MeasurementBus=off  RLa="[Ra  0.002]"  RLf=[0.0054 0.0125]  Laf=Laf  MachineConstant=Torque constant (N.m/A)  Ke=1.8  Kt=1.8  J=137  Bm=0  Tf=0  w0=w_initial  Ifinit=0  TsPowergui=0  TsBlock=-1
  Voltage Measurement2 : spsVoltageMeasurementLib/Voltage Measurement  PhasorSimulation=off  OutputType=Complex  PSBequivalent=0
  A+ : PMIOPort  Side=Left
  A- : PMIOPort  Port=2  Side=Left
  Measurement : Outport
  Va : Outport  Port=2
  wires:
  DC Machine1/1 -> Measurement/1
  Vf/1 -> Controlled Voltage Source1/1
  Voltage Measurement2/1 -> Va/1  "Armature Voltage"
  connections:
  Voltage Measurement2/LConn1 -- A+/RConn1 -- DC Machine1/LConn1
  A-/RConn1 -- Voltage Measurement2/LConn2 -- DC Machine1/RConn1
  DC Machine1/LConn2 -- Controlled Voltage Source1/RConn1
  DC Machine1/RConn2 -- Controlled Voltage Source1/LConn1

== system HSX_PPS_series0226_2/Subsystem1/DC Gen15 ==
  Vf : Inport
  Controlled Voltage Source1 : spsControlledVoltageSourceLib/Controlled Voltage Source  Initialize=on  Source_Type=DC  Amplitude=0  Phase=0  Frequency=0  Measurements=Voltage
  DC Machine1 : spsDCMachineLib/DC Machine  PresetModel=No  MechanicalLoad=Torque TL  FieldType=Wound  ShowDetailedParameters=on  MeasurementBus=off  RLa="[Ra  0.002]"  RLf=[0.0054 0.0125]  Laf=Laf  MachineConstant=Torque constant (N.m/A)  Ke=1.8  Kt=1.8  J=137  Bm=0  Tf=0  w0=w_initial  Ifinit=0  TsPowergui=0  TsBlock=-1
  Voltage Measurement2 : spsVoltageMeasurementLib/Voltage Measurement  PhasorSimulation=off  OutputType=Complex  PSBequivalent=0
  A+ : PMIOPort  Side=Left
  A- : PMIOPort  Port=2  Side=Left
  Measurement : Outport
  Va : Outport  Port=2
  wires:
  DC Machine1/1 -> Measurement/1
  Vf/1 -> Controlled Voltage Source1/1
  Voltage Measurement2/1 -> Va/1  "Armature Voltage"
  connections:
  Voltage Measurement2/LConn1 -- A+/RConn1 -- DC Machine1/LConn1
  A-/RConn1 -- Voltage Measurement2/LConn2 -- DC Machine1/RConn1
  DC Machine1/LConn2 -- Controlled Voltage Source1/RConn1
  DC Machine1/RConn2 -- Controlled Voltage Source1/LConn1

== system HSX_PPS_series0226_2/Subsystem1/DC Gen2 ==
  Vf : Inport
  Controlled Voltage Source1 : spsControlledVoltageSourceLib/Controlled Voltage Source  Initialize=on  Source_Type=DC  Amplitude=0  Phase=0  Frequency=0  Measurements=Voltage
  DC Machine1 : spsDCMachineLib/DC Machine  PresetModel=No  MechanicalLoad=Torque TL  FieldType=Wound  ShowDetailedParameters=on  MeasurementBus=off  RLa="[Ra  0.002]"  RLf=[0.0054 0.0125]  Laf=Laf  MachineConstant=Torque constant (N.m/A)  Ke=1.8  Kt=1.8  J=137  Bm=0  Tf=0  w0=w_initial  Ifinit=0  TsPowergui=0  TsBlock=-1
  Voltage Measurement2 : spsVoltageMeasurementLib/Voltage Measurement  PhasorSimulation=off  OutputType=Complex  PSBequivalent=0
  A+ : PMIOPort  Side=Left
  A- : PMIOPort  Port=2  Side=Left
  Measurement : Outport
  Va : Outport  Port=2
  wires:
  DC Machine1/1 -> Measurement/1
  Vf/1 -> Controlled Voltage Source1/1
  Voltage Measurement2/1 -> Va/1  "Armature Voltage"
  connections:
  Voltage Measurement2/LConn1 -- A+/RConn1 -- DC Machine1/LConn1
  A-/RConn1 -- Voltage Measurement2/LConn2 -- DC Machine1/RConn1
  DC Machine1/LConn2 -- Controlled Voltage Source1/RConn1
  DC Machine1/RConn2 -- Controlled Voltage Source1/LConn1

== system HSX_PPS_series0226_2/Subsystem1/DC Gen3 ==
  Vf : Inport
  Controlled Voltage Source1 : spsControlledVoltageSourceLib/Controlled Voltage Source  Initialize=on  Source_Type=DC  Amplitude=0  Phase=0  Frequency=0  Measurements=Voltage
  DC Machine1 : spsDCMachineLib/DC Machine  PresetModel=No  MechanicalLoad=Torque TL  FieldType=Wound  ShowDetailedParameters=on  MeasurementBus=off  RLa="[Ra  0.002]"  RLf=[0.0054 0.0125]  Laf=Laf  MachineConstant=Torque constant (N.m/A)  Ke=1.8  Kt=1.8  J=137  Bm=0  Tf=0  w0=w_initial  Ifinit=0  TsPowergui=0  TsBlock=-1
  Voltage Measurement2 : spsVoltageMeasurementLib/Voltage Measurement  PhasorSimulation=off  OutputType=Complex  PSBequivalent=0
  A+ : PMIOPort  Side=Left
  A- : PMIOPort  Port=2  Side=Left
  Measurement : Outport
  Va : Outport  Port=2
  wires:
  DC Machine1/1 -> Measurement/1
  Vf/1 -> Controlled Voltage Source1/1
  Voltage Measurement2/1 -> Va/1  "Armature Voltage"
  connections:
  Voltage Measurement2/LConn1 -- A+/RConn1 -- DC Machine1/LConn1
  A-/RConn1 -- Voltage Measurement2/LConn2 -- DC Machine1/RConn1
  DC Machine1/LConn2 -- Controlled Voltage Source1/RConn1
  DC Machine1/RConn2 -- Controlled Voltage Source1/LConn1

== system HSX_PPS_series0226_2/Subsystem1/DC Gen4 ==
  Vf : Inport
  Controlled Voltage Source1 : spsControlledVoltageSourceLib/Controlled Voltage Source  Initialize=on  Source_Type=DC  Amplitude=0  Phase=0  Frequency=0  Measurements=Voltage
  DC Machine1 : spsDCMachineLib/DC Machine  PresetModel=No  MechanicalLoad=Torque TL  FieldType=Wound  ShowDetailedParameters=on  MeasurementBus=off  RLa="[Ra  0.002]"  RLf=[0.0054 0.0125]  Laf=Laf  MachineConstant=Torque constant (N.m/A)  Ke=1.8  Kt=1.8  J=137  Bm=0  Tf=0  w0=w_initial  Ifinit=0  TsPowergui=0  TsBlock=-1
  Voltage Measurement2 : spsVoltageMeasurementLib/Voltage Measurement  PhasorSimulation=off  OutputType=Complex  PSBequivalent=0
  A+ : PMIOPort  Side=Left
  A- : PMIOPort  Port=2  Side=Left
  Measurement : Outport
  Va : Outport  Port=2
  wires:
  DC Machine1/1 -> Measurement/1
  Vf/1 -> Controlled Voltage Source1/1
  Voltage Measurement2/1 -> Va/1  "Armature Voltage"
  connections:
  Voltage Measurement2/LConn1 -- A+/RConn1 -- DC Machine1/LConn1
  A-/RConn1 -- Voltage Measurement2/LConn2 -- DC Machine1/RConn1
  DC Machine1/LConn2 -- Controlled Voltage Source1/RConn1
  DC Machine1/RConn2 -- Controlled Voltage Source1/LConn1

== system HSX_PPS_series0226_2/Subsystem1/DC Gen5 ==
  Vf : Inport
  Controlled Voltage Source1 : spsControlledVoltageSourceLib/Controlled Voltage Source  Initialize=on  Source_Type=DC  Amplitude=0  Phase=0  Frequency=0  Measurements=Voltage
  DC Machine1 : spsDCMachineLib/DC Machine  PresetModel=No  MechanicalLoad=Torque TL  FieldType=Wound  ShowDetailedParameters=on  MeasurementBus=off  RLa="[Ra  0.002]"  RLf=[0.0054 0.0125]  Laf=Laf  MachineConstant=Torque constant (N.m/A)  Ke=1.8  Kt=1.8  J=137  Bm=0  Tf=0  w0=w_initial  Ifinit=0  TsPowergui=0  TsBlock=-1
  Voltage Measurement2 : spsVoltageMeasurementLib/Voltage Measurement  PhasorSimulation=off  OutputType=Complex  PSBequivalent=0
  A+ : PMIOPort  Side=Left
  A- : PMIOPort  Port=2  Side=Left
  Measurement : Outport
  Va : Outport  Port=2
  wires:
  DC Machine1/1 -> Measurement/1
  Vf/1 -> Controlled Voltage Source1/1
  Voltage Measurement2/1 -> Va/1  "Armature Voltage"
  connections:
  Voltage Measurement2/LConn1 -- A+/RConn1 -- DC Machine1/LConn1
  A-/RConn1 -- Voltage Measurement2/LConn2 -- DC Machine1/RConn1
  DC Machine1/LConn2 -- Controlled Voltage Source1/RConn1
  DC Machine1/RConn2 -- Controlled Voltage Source1/LConn1

== system HSX_PPS_series0226_2/Subsystem1/DC Gen6 ==
  Vf : Inport
  Controlled Voltage Source1 : spsControlledVoltageSourceLib/Controlled Voltage Source  Initialize=on  Source_Type=DC  Amplitude=0  Phase=0  Frequency=0  Measurements=Voltage
  DC Machine1 : spsDCMachineLib/DC Machine  PresetModel=No  MechanicalLoad=Torque TL  FieldType=Wound  ShowDetailedParameters=on  MeasurementBus=off  RLa="[Ra  0.002]"  RLf=[0.0054 0.0125]  Laf=Laf  MachineConstant=Torque constant (N.m/A)  Ke=1.8  Kt=1.8  J=137  Bm=0  Tf=0  w0=w_initial  Ifinit=0  TsPowergui=0  TsBlock=-1
  Voltage Measurement2 : spsVoltageMeasurementLib/Voltage Measurement  PhasorSimulation=off  OutputType=Complex  PSBequivalent=0
  A+ : PMIOPort  Side=Left
  A- : PMIOPort  Port=2  Side=Left
  Measurement : Outport
  Va : Outport  Port=2
  wires:
  DC Machine1/1 -> Measurement/1
  Vf/1 -> Controlled Voltage Source1/1
  Voltage Measurement2/1 -> Va/1  "Armature Voltage"
  connections:
  Voltage Measurement2/LConn1 -- A+/RConn1 -- DC Machine1/LConn1
  A-/RConn1 -- Voltage Measurement2/LConn2 -- DC Machine1/RConn1
  DC Machine1/LConn2 -- Controlled Voltage Source1/RConn1
  DC Machine1/RConn2 -- Controlled Voltage Source1/LConn1

== system HSX_PPS_series0226_2/Subsystem1/DC Gen7 ==
  Vf : Inport
  Controlled Voltage Source1 : spsControlledVoltageSourceLib/Controlled Voltage Source  Initialize=on  Source_Type=DC  Amplitude=0  Phase=0  Frequency=0  Measurements=Voltage
  DC Machine1 : spsDCMachineLib/DC Machine  PresetModel=No  MechanicalLoad=Torque TL  FieldType=Wound  ShowDetailedParameters=on  MeasurementBus=off  RLa="[Ra  0.002]"  RLf=[0.0054 0.0125]  Laf=Laf  MachineConstant=Torque constant (N.m/A)  Ke=1.8  Kt=1.8  J=137  Bm=0  Tf=0  w0=w_initial  Ifinit=0  TsPowergui=0  TsBlock=-1
  Voltage Measurement2 : spsVoltageMeasurementLib/Voltage Measurement  PhasorSimulation=off  OutputType=Complex  PSBequivalent=0
  A+ : PMIOPort  Side=Left
  A- : PMIOPort  Port=2  Side=Left
  Measurement : Outport
  Va : Outport  Port=2
  wires:
  DC Machine1/1 -> Measurement/1
  Vf/1 -> Controlled Voltage Source1/1
  Voltage Measurement2/1 -> Va/1  "Armature Voltage"
  connections:
  Voltage Measurement2/LConn1 -- A+/RConn1 -- DC Machine1/LConn1
  A-/RConn1 -- Voltage Measurement2/LConn2 -- DC Machine1/RConn1
  DC Machine1/LConn2 -- Controlled Voltage Source1/RConn1
  DC Machine1/RConn2 -- Controlled Voltage Source1/LConn1

== system HSX_PPS_series0226_2/Subsystem1/DC Gen8 ==
  Vf : Inport
  Controlled Voltage Source1 : spsControlledVoltageSourceLib/Controlled Voltage Source  Initialize=on  Source_Type=DC  Amplitude=0  Phase=0  Frequency=0  Measurements=Voltage
  DC Machine1 : spsDCMachineLib/DC Machine  PresetModel=No  MechanicalLoad=Torque TL  FieldType=Wound  ShowDetailedParameters=on  MeasurementBus=off  RLa="[Ra  0.002]"  RLf=[0.0054 0.0125]  Laf=Laf  MachineConstant=Torque constant (N.m/A)  Ke=1.8  Kt=1.8  J=137  Bm=0  Tf=0  w0=w_initial  Ifinit=0  TsPowergui=0  TsBlock=-1
  Voltage Measurement2 : spsVoltageMeasurementLib/Voltage Measurement  PhasorSimulation=off  OutputType=Complex  PSBequivalent=0
  A+ : PMIOPort  Side=Left
  A- : PMIOPort  Port=2  Side=Left
  Measurement : Outport
  Va : Outport  Port=2
  wires:
  DC Machine1/1 -> Measurement/1
  Vf/1 -> Controlled Voltage Source1/1
  Voltage Measurement2/1 -> Va/1  "Armature Voltage"
  connections:
  Voltage Measurement2/LConn1 -- A+/RConn1 -- DC Machine1/LConn1
  A-/RConn1 -- Voltage Measurement2/LConn2 -- DC Machine1/RConn1
  DC Machine1/LConn2 -- Controlled Voltage Source1/RConn1
  DC Machine1/RConn2 -- Controlled Voltage Source1/LConn1

== system HSX_PPS_series0226_2/Subsystem1/DC Gen9 ==
  Vf : Inport
  Controlled Voltage Source1 : spsControlledVoltageSourceLib/Controlled Voltage Source  Initialize=on  Source_Type=DC  Amplitude=0  Phase=0  Frequency=0  Measurements=Voltage
  DC Machine1 : spsDCMachineLib/DC Machine  PresetModel=No  MechanicalLoad=Torque TL  FieldType=Wound  ShowDetailedParameters=on  MeasurementBus=off  RLa="[Ra  0.002]"  RLf=[0.0054 0.0125]  Laf=Laf  MachineConstant=Torque constant (N.m/A)  Ke=1.8  Kt=1.8  J=137  Bm=0  Tf=0  w0=w_initial  Ifinit=0  TsPowergui=0  TsBlock=-1
  Voltage Measurement2 : spsVoltageMeasurementLib/Voltage Measurement  PhasorSimulation=off  OutputType=Complex  PSBequivalent=0
  A+ : PMIOPort  Side=Left
  A- : PMIOPort  Port=2  Side=Left
  Measurement : Outport
  Va : Outport  Port=2
  wires:
  DC Machine1/1 -> Measurement/1
  Vf/1 -> Controlled Voltage Source1/1
  Voltage Measurement2/1 -> Va/1  "Armature Voltage"
  connections:
  Voltage Measurement2/LConn1 -- A+/RConn1 -- DC Machine1/LConn1
  A-/RConn1 -- Voltage Measurement2/LConn2 -- DC Machine1/RConn1
  DC Machine1/LConn2 -- Controlled Voltage Source1/RConn1
  DC Machine1/RConn2 -- Controlled Voltage Source1/LConn1

== system HSX_PPS_series0226_2/Subsystem2/DC Gen ==
  Vf : Inport
  Controlled Voltage Source1 : spsControlledVoltageSourceLib/Controlled Voltage Source  Initialize=on  Source_Type=DC  Amplitude=0  Phase=0  Frequency=0  Measurements=Voltage
  DC Machine1 : spsDCMachineLib/DC Machine  PresetModel=No  MechanicalLoad=Torque TL  FieldType=Wound  ShowDetailedParameters=on  MeasurementBus=off  RLa="[Ra  0.002]"  RLf=[0.0054 0.0125]  Laf=Laf  MachineConstant=Torque constant (N.m/A)  Ke=1.8  Kt=1.8  J=137  Bm=0  Tf=0  w0=w_initial  Ifinit=0  TsPowergui=0  TsBlock=-1
  Voltage Measurement2 : spsVoltageMeasurementLib/Voltage Measurement  PhasorSimulation=off  OutputType=Complex  PSBequivalent=0
  A+ : PMIOPort  Side=Left
  A- : PMIOPort  Port=2  Side=Left
  Measurement : Outport
  Va : Outport  Port=2
  wires:
  DC Machine1/1 -> Measurement/1
  Vf/1 -> Controlled Voltage Source1/1
  Voltage Measurement2/1 -> Va/1  "Armature Voltage"
  connections:
  Voltage Measurement2/LConn1 -- A+/RConn1 -- DC Machine1/LConn1
  A-/RConn1 -- Voltage Measurement2/LConn2 -- DC Machine1/RConn1
  DC Machine1/LConn2 -- Controlled Voltage Source1/RConn1
  DC Machine1/RConn2 -- Controlled Voltage Source1/LConn1

== system HSX_PPS_series0226_2/Subsystem2/DC Gen1 ==
  Vf : Inport
  Controlled Voltage Source1 : spsControlledVoltageSourceLib/Controlled Voltage Source  Initialize=on  Source_Type=DC  Amplitude=0  Phase=0  Frequency=0  Measurements=Voltage
  DC Machine1 : spsDCMachineLib/DC Machine  PresetModel=No  MechanicalLoad=Torque TL  FieldType=Wound  ShowDetailedParameters=on  MeasurementBus=off  RLa="[Ra  0.002]"  RLf=[0.0054 0.0125]  Laf=Laf  MachineConstant=Torque constant (N.m/A)  Ke=1.8  Kt=1.8  J=137  Bm=0  Tf=0  w0=w_initial  Ifinit=0  TsPowergui=0  TsBlock=-1
  Voltage Measurement2 : spsVoltageMeasurementLib/Voltage Measurement  PhasorSimulation=off  OutputType=Complex  PSBequivalent=0
  A+ : PMIOPort  Side=Left
  A- : PMIOPort  Port=2  Side=Left
  Measurement : Outport
  Va : Outport  Port=2
  wires:
  DC Machine1/1 -> Measurement/1
  Vf/1 -> Controlled Voltage Source1/1
  Voltage Measurement2/1 -> Va/1  "Armature Voltage"
  connections:
  Voltage Measurement2/LConn1 -- A+/RConn1 -- DC Machine1/LConn1
  A-/RConn1 -- Voltage Measurement2/LConn2 -- DC Machine1/RConn1
  DC Machine1/LConn2 -- Controlled Voltage Source1/RConn1
  DC Machine1/RConn2 -- Controlled Voltage Source1/LConn1

== system HSX_PPS_series0226_2/Subsystem2/DC Gen10 ==
  Vf : Inport
  Controlled Voltage Source1 : spsControlledVoltageSourceLib/Controlled Voltage Source  Initialize=on  Source_Type=DC  Amplitude=0  Phase=0  Frequency=0  Measurements=Voltage
  DC Machine1 : spsDCMachineLib/DC Machine  PresetModel=No  MechanicalLoad=Torque TL  FieldType=Wound  ShowDetailedParameters=on  MeasurementBus=off  RLa="[Ra  0.002]"  RLf=[0.0054 0.0125]  Laf=Laf  MachineConstant=Torque constant (N.m/A)  Ke=1.8  Kt=1.8  J=137  Bm=0  Tf=0  w0=w_initial  Ifinit=0  TsPowergui=0  TsBlock=-1
  Voltage Measurement2 : spsVoltageMeasurementLib/Voltage Measurement  PhasorSimulation=off  OutputType=Complex  PSBequivalent=0
  A+ : PMIOPort  Side=Left
  A- : PMIOPort  Port=2  Side=Left
  Measurement : Outport
  Va : Outport  Port=2
  wires:
  DC Machine1/1 -> Measurement/1
  Vf/1 -> Controlled Voltage Source1/1
  Voltage Measurement2/1 -> Va/1  "Armature Voltage"
  connections:
  Voltage Measurement2/LConn1 -- A+/RConn1 -- DC Machine1/LConn1
  A-/RConn1 -- Voltage Measurement2/LConn2 -- DC Machine1/RConn1
  DC Machine1/LConn2 -- Controlled Voltage Source1/RConn1
  DC Machine1/RConn2 -- Controlled Voltage Source1/LConn1

== system HSX_PPS_series0226_2/Subsystem2/DC Gen11 ==
  Vf : Inport
  Controlled Voltage Source1 : spsControlledVoltageSourceLib/Controlled Voltage Source  Initialize=on  Source_Type=DC  Amplitude=0  Phase=0  Frequency=0  Measurements=Voltage
  DC Machine1 : spsDCMachineLib/DC Machine  PresetModel=No  MechanicalLoad=Torque TL  FieldType=Wound  ShowDetailedParameters=on  MeasurementBus=off  RLa="[Ra  0.002]"  RLf=[0.0054 0.0125]  Laf=Laf  MachineConstant=Torque constant (N.m/A)  Ke=1.8  Kt=1.8  J=137  Bm=0  Tf=0  w0=w_initial  Ifinit=0  TsPowergui=0  TsBlock=-1
  Voltage Measurement2 : spsVoltageMeasurementLib/Voltage Measurement  PhasorSimulation=off  OutputType=Complex  PSBequivalent=0
  A+ : PMIOPort  Side=Left
  A- : PMIOPort  Port=2  Side=Left
  Measurement : Outport
  Va : Outport  Port=2
  wires:
  DC Machine1/1 -> Measurement/1
  Vf/1 -> Controlled Voltage Source1/1
  Voltage Measurement2/1 -> Va/1  "Armature Voltage"
  connections:
  Voltage Measurement2/LConn1 -- A+/RConn1 -- DC Machine1/LConn1
  A-/RConn1 -- Voltage Measurement2/LConn2 -- DC Machine1/RConn1
  DC Machine1/LConn2 -- Controlled Voltage Source1/RConn1
  DC Machine1/RConn2 -- Controlled Voltage Source1/LConn1

== system HSX_PPS_series0226_2/Subsystem2/DC Gen12 ==
  Vf : Inport
  Controlled Voltage Source1 : spsControlledVoltageSourceLib/Controlled Voltage Source  Initialize=on  Source_Type=DC  Amplitude=0  Phase=0  Frequency=0  Measurements=Voltage
  DC Machine1 : spsDCMachineLib/DC Machine  PresetModel=No  MechanicalLoad=Torque TL  FieldType=Wound  ShowDetailedParameters=on  MeasurementBus=off  RLa="[Ra  0.002]"  RLf=[0.0054 0.0125]  Laf=Laf  MachineConstant=Torque constant (N.m/A)  Ke=1.8  Kt=1.8  J=137  Bm=0  Tf=0  w0=w_initial  Ifinit=0  TsPowergui=0  TsBlock=-1
  Voltage Measurement2 : spsVoltageMeasurementLib/Voltage Measurement  PhasorSimulation=off  OutputType=Complex  PSBequivalent=0
  A+ : PMIOPort  Side=Left
  A- : PMIOPort  Port=2  Side=Left
  Measurement : Outport
  Va : Outport  Port=2
  wires:
  DC Machine1/1 -> Measurement/1
  Vf/1 -> Controlled Voltage Source1/1
  Voltage Measurement2/1 -> Va/1  "Armature Voltage"
  connections:
  Voltage Measurement2/LConn1 -- A+/RConn1 -- DC Machine1/LConn1
  A-/RConn1 -- Voltage Measurement2/LConn2 -- DC Machine1/RConn1
  DC Machine1/LConn2 -- Controlled Voltage Source1/RConn1
  DC Machine1/RConn2 -- Controlled Voltage Source1/LConn1

== system HSX_PPS_series0226_2/Subsystem2/DC Gen13 ==
  Vf : Inport
  Controlled Voltage Source1 : spsControlledVoltageSourceLib/Controlled Voltage Source  Initialize=on  Source_Type=DC  Amplitude=0  Phase=0  Frequency=0  Measurements=Voltage
  DC Machine1 : spsDCMachineLib/DC Machine  PresetModel=No  MechanicalLoad=Torque TL  FieldType=Wound  ShowDetailedParameters=on  MeasurementBus=off  RLa="[Ra  0.002]"  RLf=[0.0054 0.0125]  Laf=Laf  MachineConstant=Torque constant (N.m/A)  Ke=1.8  Kt=1.8  J=137  Bm=0  Tf=0  w0=w_initial  Ifinit=0  TsPowergui=0  TsBlock=-1
  Voltage Measurement2 : spsVoltageMeasurementLib/Voltage Measurement  PhasorSimulation=off  OutputType=Complex  PSBequivalent=0
  A+ : PMIOPort  Side=Left
  A- : PMIOPort  Port=2  Side=Left
  Measurement : Outport
  Va : Outport  Port=2
  wires:
  DC Machine1/1 -> Measurement/1
  Vf/1 -> Controlled Voltage Source1/1
  Voltage Measurement2/1 -> Va/1  "Armature Voltage"
  connections:
  Voltage Measurement2/LConn1 -- A+/RConn1 -- DC Machine1/LConn1
  A-/RConn1 -- Voltage Measurement2/LConn2 -- DC Machine1/RConn1
  DC Machine1/LConn2 -- Controlled Voltage Source1/RConn1
  DC Machine1/RConn2 -- Controlled Voltage Source1/LConn1

== system HSX_PPS_series0226_2/Subsystem2/DC Gen14 ==
  Vf : Inport
  Controlled Voltage Source1 : spsControlledVoltageSourceLib/Controlled Voltage Source  Initialize=on  Source_Type=DC  Amplitude=0  Phase=0  Frequency=0  Measurements=Voltage
  DC Machine1 : spsDCMachineLib/DC Machine  PresetModel=No  MechanicalLoad=Torque TL  FieldType=Wound  ShowDetailedParameters=on  MeasurementBus=off  RLa="[Ra  0.002]"  RLf=[0.0054 0.0125]  Laf=Laf  MachineConstant=Torque constant (N.m/A)  Ke=1.8  Kt=1.8  J=137  Bm=0  Tf=0  w0=w_initial  Ifinit=0  TsPowergui=0  TsBlock=-1
  Voltage Measurement2 : spsVoltageMeasurementLib/Voltage Measurement  PhasorSimulation=off  OutputType=Complex  PSBequivalent=0
  A+ : PMIOPort  Side=Left
  A- : PMIOPort  Port=2  Side=Left
  Measurement : Outport
  Va : Outport  Port=2
  wires:
  DC Machine1/1 -> Measurement/1
  Vf/1 -> Controlled Voltage Source1/1
  Voltage Measurement2/1 -> Va/1  "Armature Voltage"
  connections:
  Voltage Measurement2/LConn1 -- A+/RConn1 -- DC Machine1/LConn1
  A-/RConn1 -- Voltage Measurement2/LConn2 -- DC Machine1/RConn1
  DC Machine1/LConn2 -- Controlled Voltage Source1/RConn1
  DC Machine1/RConn2 -- Controlled Voltage Source1/LConn1

== system HSX_PPS_series0226_2/Subsystem2/DC Gen15 ==
  Vf : Inport
  Controlled Voltage Source1 : spsControlledVoltageSourceLib/Controlled Voltage Source  Initialize=on  Source_Type=DC  Amplitude=0  Phase=0  Frequency=0  Measurements=Voltage
  DC Machine1 : spsDCMachineLib/DC Machine  PresetModel=No  MechanicalLoad=Torque TL  FieldType=Wound  ShowDetailedParameters=on  MeasurementBus=off  RLa="[Ra  0.002]"  RLf=[0.0054 0.0125]  Laf=Laf  MachineConstant=Torque constant (N.m/A)  Ke=1.8  Kt=1.8  J=137  Bm=0  Tf=0  w0=w_initial  Ifinit=0  TsPowergui=0  TsBlock=-1
  Voltage Measurement2 : spsVoltageMeasurementLib/Voltage Measurement  PhasorSimulation=off  OutputType=Complex  PSBequivalent=0
  A+ : PMIOPort  Side=Left
  A- : PMIOPort  Port=2  Side=Left
  Measurement : Outport
  Va : Outport  Port=2
  wires:
  DC Machine1/1 -> Measurement/1
  Vf/1 -> Controlled Voltage Source1/1
  Voltage Measurement2/1 -> Va/1  "Armature Voltage"
  connections:
  Voltage Measurement2/LConn1 -- A+/RConn1 -- DC Machine1/LConn1
  A-/RConn1 -- Voltage Measurement2/LConn2 -- DC Machine1/RConn1
  DC Machine1/LConn2 -- Controlled Voltage Source1/RConn1
  DC Machine1/RConn2 -- Controlled Voltage Source1/LConn1

== system HSX_PPS_series0226_2/Subsystem2/DC Gen2 ==
  Vf : Inport
  Controlled Voltage Source1 : spsControlledVoltageSourceLib/Controlled Voltage Source  Initialize=on  Source_Type=DC  Amplitude=0  Phase=0  Frequency=0  Measurements=Voltage
  DC Machine1 : spsDCMachineLib/DC Machine  PresetModel=No  MechanicalLoad=Torque TL  FieldType=Wound  ShowDetailedParameters=on  MeasurementBus=off  RLa="[Ra  0.002]"  RLf=[0.0054 0.0125]  Laf=Laf  MachineConstant=Torque constant (N.m/A)  Ke=1.8  Kt=1.8  J=137  Bm=0  Tf=0  w0=w_initial  Ifinit=0  TsPowergui=0  TsBlock=-1
  Voltage Measurement2 : spsVoltageMeasurementLib/Voltage Measurement  PhasorSimulation=off  OutputType=Complex  PSBequivalent=0
  A+ : PMIOPort  Side=Left
  A- : PMIOPort  Port=2  Side=Left
  Measurement : Outport
  Va : Outport  Port=2
  wires:
  DC Machine1/1 -> Measurement/1
  Vf/1 -> Controlled Voltage Source1/1
  Voltage Measurement2/1 -> Va/1  "Armature Voltage"
  connections:
  Voltage Measurement2/LConn1 -- A+/RConn1 -- DC Machine1/LConn1
  A-/RConn1 -- Voltage Measurement2/LConn2 -- DC Machine1/RConn1
  DC Machine1/LConn2 -- Controlled Voltage Source1/RConn1
  DC Machine1/RConn2 -- Controlled Voltage Source1/LConn1

== system HSX_PPS_series0226_2/Subsystem2/DC Gen3 ==
  Vf : Inport
  Controlled Voltage Source1 : spsControlledVoltageSourceLib/Controlled Voltage Source  Initialize=on  Source_Type=DC  Amplitude=0  Phase=0  Frequency=0  Measurements=Voltage
  DC Machine1 : spsDCMachineLib/DC Machine  PresetModel=No  MechanicalLoad=Torque TL  FieldType=Wound  ShowDetailedParameters=on  MeasurementBus=off  RLa="[Ra  0.002]"  RLf=[0.0054 0.0125]  Laf=Laf  MachineConstant=Torque constant (N.m/A)  Ke=1.8  Kt=1.8  J=137  Bm=0  Tf=0  w0=w_initial  Ifinit=0  TsPowergui=0  TsBlock=-1
  Voltage Measurement2 : spsVoltageMeasurementLib/Voltage Measurement  PhasorSimulation=off  OutputType=Complex  PSBequivalent=0
  A+ : PMIOPort  Side=Left
  A- : PMIOPort  Port=2  Side=Left
  Measurement : Outport
  Va : Outport  Port=2
  wires:
  DC Machine1/1 -> Measurement/1
  Vf/1 -> Controlled Voltage Source1/1
  Voltage Measurement2/1 -> Va/1  "Armature Voltage"
  connections:
  Voltage Measurement2/LConn1 -- A+/RConn1 -- DC Machine1/LConn1
  A-/RConn1 -- Voltage Measurement2/LConn2 -- DC Machine1/RConn1
  DC Machine1/LConn2 -- Controlled Voltage Source1/RConn1
  DC Machine1/RConn2 -- Controlled Voltage Source1/LConn1

== system HSX_PPS_series0226_2/Subsystem2/DC Gen4 ==
  Vf : Inport
  Controlled Voltage Source1 : spsControlledVoltageSourceLib/Controlled Voltage Source  Initialize=on  Source_Type=DC  Amplitude=0  Phase=0  Frequency=0  Measurements=Voltage
  DC Machine1 : spsDCMachineLib/DC Machine  PresetModel=No  MechanicalLoad=Torque TL  FieldType=Wound  ShowDetailedParameters=on  MeasurementBus=off  RLa="[Ra  0.002]"  RLf=[0.0054 0.0125]  Laf=Laf  MachineConstant=Torque constant (N.m/A)  Ke=1.8  Kt=1.8  J=137  Bm=0  Tf=0  w0=w_initial  Ifinit=0  TsPowergui=0  TsBlock=-1
  Voltage Measurement2 : spsVoltageMeasurementLib/Voltage Measurement  PhasorSimulation=off  OutputType=Complex  PSBequivalent=0
  A+ : PMIOPort  Side=Left
  A- : PMIOPort  Port=2  Side=Left
  Measurement : Outport
  Va : Outport  Port=2
  wires:
  DC Machine1/1 -> Measurement/1
  Vf/1 -> Controlled Voltage Source1/1
  Voltage Measurement2/1 -> Va/1  "Armature Voltage"
  connections:
  Voltage Measurement2/LConn1 -- A+/RConn1 -- DC Machine1/LConn1
  A-/RConn1 -- Voltage Measurement2/LConn2 -- DC Machine1/RConn1
  DC Machine1/LConn2 -- Controlled Voltage Source1/RConn1
  DC Machine1/RConn2 -- Controlled Voltage Source1/LConn1
